simulink model "CommandePontComplet"  (R2025a)
settings: Solver=ode23t  StartTime=0.0  StopTime=5  RelTol=1e-3
libraries: spsSeriesRLCBranchLib x7, spsDiodeLib x4, spsMosfetLib x4, spsDCVoltageSourceLib x2, spsCurrentMeasurementLib x1, spsLinearTransformerLib x1, spsVoltageMeasurementLib x1, sps_lib x1
settings Model: Creator=logar  LastModifiedBy=hassan

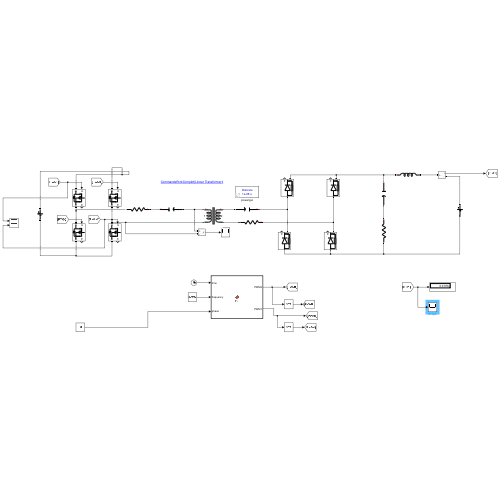
[thumbnail: Simulink's stored preview of the top-level diagram]
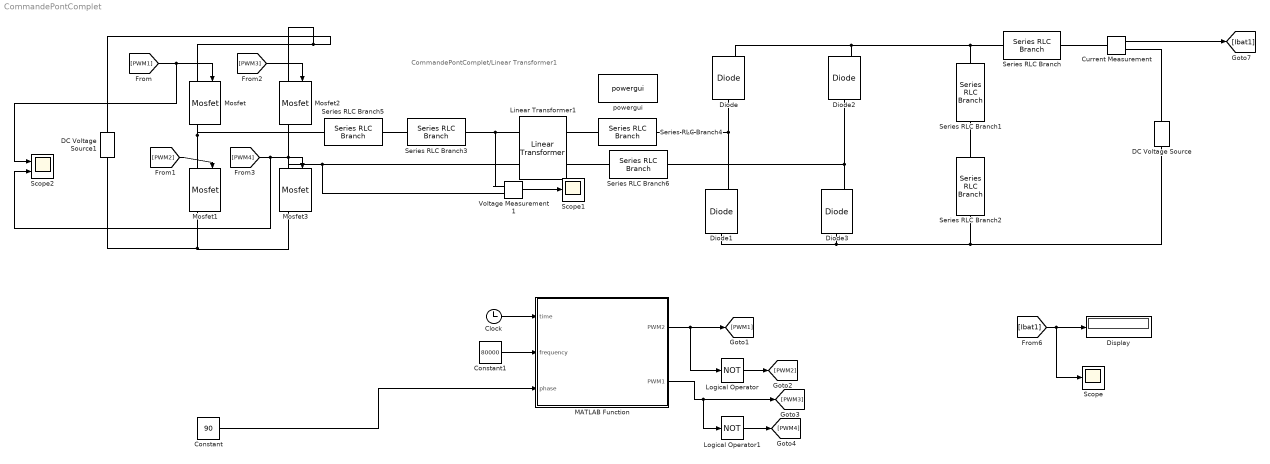
== system CommandePontComplet ==
  note: CommandePontComplet/Linear Transformer1
  Clock : Clock
  Constant : Constant  Value=90
  Constant1 : Constant  Value=80000
  Current Measurement : spsCurrentMeasurementLib/Current Measurement  PhasorSimulation=off  OutputType=Complex  PSBequivalent=0
  DC Voltage Source : spsDCVoltageSourceLib/DC Voltage Source  Amplitude=48  Measurements=None
  DC Voltage Source1 : spsDCVoltageSourceLib/DC Voltage Source  Amplitude=400  Measurements=None
  Diode{,1..3} (4 alike) : spsDiodeLib/Diode  Ron=0.001  Lon=0  Vf=0.8  IC=0  UseSnubber=0  Rs=500  Cs=250e-9  Measurements=on
  Display : Display
  Linear Transformer1 : spsLinearTransformerLib/Linear Transformer  UNITS=SI  NominalPower=[ 2000 80e3 ]  winding1=[400 4.3218e-09 0.00089501]  winding2=[70 7.938e-10 0.000338]  ThreeWindings=off  winding3=[3.15e+05 0.7938 0.084225]  RmLm=[1.0805e+06 2866.1]  Measurements=None  DataType=on
  Logical Operator : Logic  Operator=NOT  AllPortsSameDT=off  OutDataTypeStr=boolean
  Logical Operator1 : Logic  Operator=NOT  AllPortsSameDT=off  OutDataTypeStr=boolean
  MATLAB Function : MATLAB Function  TreatAsAtomicUnit=on
  Mosfet{,1..3} (4 alike) : spsMosfetLib/Mosfet  Ron=0.1  Lon=0  Rd=0.01  Vfd=0  IC=0  Rs=1e5  Cs=inf  Measurements=on
  Scope : Scope
      settings: ActiveDisplayYMinimum=-0.00099507474157943879  ActiveDisplayYMaximum=0.040324566346598756
  Scope1 : Scope
      settings: ActiveDisplayYMinimum=-402.56471596665705  ActiveDisplayYMaximum=404.97381059399561
  Scope2 : Scope  NumInputPorts=2
      settings: ActiveDisplayYMinimum=-0.025124580830577781  ActiveDisplayYMaximum=1.019798521825793  DataLoggingVariableName=ScopeData2
  Series RLC Branch : spsSeriesRLCBranchLib/Series RLC Branch  LConnTagsString=__new0  RConnTagsString=__new0  BranchType=L  Resistance=1  Inductance=40e-6  SetiL0=off  InitialCurrent=0  Capacitance=1e-6  Setx0=off  InitialVoltage=0  Measurements=None
  Series RLC Branch1 : spsSeriesRLCBranchLib/Series RLC Branch  LConnTagsString=__new0  RConnTagsString=__new0  BranchType=C  Resistance=1  Inductance=1e-3  SetiL0=off  InitialCurrent=0  Capacitance=200e-6  Setx0=off  InitialVoltage=0  Measurements=None
  Series RLC Branch2 : spsSeriesRLCBranchLib/Series RLC Branch  LConnTagsString=__new0  RConnTagsString=__new0  BranchType=R  Resistance=10e-3  Inductance=1e-3  SetiL0=off  InitialCurrent=0  Capacitance=1e-6  Setx0=off  InitialVoltage=0  Measurements=None
  Series RLC Branch3 : spsSeriesRLCBranchLib/Series RLC Branch  LConnTagsString=__new0  RConnTagsString=__new0  BranchType=C  Resistance=1  Inductance=1e-3  SetiL0=off  InitialCurrent=0  Capacitance=100e-6  Setx0=off  InitialVoltage=0  Measurements=None
  Series RLC Branch4 : spsSeriesRLCBranchLib/Series RLC Branch  LConnTagsString=__new0  RConnTagsString=__new0  BranchType=C  Resistance=1  Inductance=1e-3  SetiL0=off  InitialCurrent=0  Capacitance=47e-6  Setx0=off  InitialVoltage=0  Measurements=None
  Series RLC Branch5 : spsSeriesRLCBranchLib/Series RLC Branch  LConnTagsString=__new0  RConnTagsString=__new0  BranchType=R  Resistance=0.05  Inductance=1e-3  SetiL0=off  InitialCurrent=0  Capacitance=1e-6  Setx0=off  InitialVoltage=0  Measurements=None
  Series RLC Branch6 : spsSeriesRLCBranchLib/Series RLC Branch  LConnTagsString=__new0  RConnTagsString=__new0  BranchType=R  Resistance=50  Inductance=1e-3  SetiL0=off  InitialCurrent=0  Capacitance=1e-6  Setx0=off  InitialVoltage=0  Measurements=None
  Voltage Measurement1 : spsVoltageMeasurementLib/Voltage Measurement  PhasorSimulation=off  OutputType=Complex  PSBequivalent=0
  powergui : sps_lib/powergui  Priority=1  SimulationMode=Discrete  SampleTime=1e-8  frequency=60  Iterations=50  frequencyindice=0  Pbase=100e6  ErrMax=1e-4  UnitsV=kV  UnitsW=MW  buscounter=0  FunctionMessages=off  echomessages=off  EnableUseOfTLC=off  CurrentSourceSwitches=off  DisableSnubberDevices=off  DisableRonSwitches=off  DisableVfSwitches=off  DisplayEquations=off  AutomaticDiscreteSolvers=off  SolverType=Tustin/Backward Euler (TBE)  Interpol=off  ExternalGateDelay=off  methode=off  Ts=100  x0status=blocks  SPID=on  SwTol=0  HookPort=off  NonlinearTolerance=1e-4  nMaxIteration=100  ContinueOnMaxIteration=off  RestoreLinks=warning  ResistiveCurrentMeasurement=off  Frange=[0:2:500]  Ylog=off  Xlog=on  ShowGrid=off  save=off  variable=ZData  structure=0  ZoomFFT=off  StartTime=0.0  cycles=1  DisplayStyle=1  fundamental=60  FreqAxis=off  MaxFrequency=1000  frequencyindicesteady=1  RmsSteady=1  display=off
  wires:
  [PWM1] -> Scope2/1, Mosfet/1
  [PWM3] -> Mosfet2/1
  [PWM2] -> Mosfet1/1
  [PWM4] -> Scope2/2, Mosfet3/1
  Constant1/1 -> MATLAB Function/2(frequency)
  Clock/1 -> MATLAB Function/1(time)
  MATLAB Function/1(PWM2) -> Logical Operator/1, [PWM1]
  Logical Operator/1 -> [PWM2]
  MATLAB Function/2(PWM1) -> Logical Operator1/1, [PWM3]
  Logical Operator1/1 -> [PWM4]
  Voltage Measurement1/1 -> Scope1/1
  Current Measurement/1 -> [Ibat1]
  [Ibat1] -> Scope/1, Display/1
  Constant/1 -> MATLAB Function/3(phase)
  connections:
  Mosfet/RConn1 -- Series RLC Branch5/RConn1 -- Mosfet1/LConn1
  Mosfet2/RConn1 -- Linear Transformer1/LConn2 -- Voltage Measurement1/LConn2 -- Mosfet3/LConn1
  Mosfet2/LConn1 -- Mosfet/LConn1 -- DC Voltage Source1/RConn1
  Mosfet3/RConn1 -- DC Voltage Source1/LConn1 -- Mosfet1/RConn1
  Diode1/RConn1 -- Series RLC Branch4/LConn1 -- Diode/LConn1
  Diode3/RConn1 -- Diode2/LConn1 -- Series RLC Branch6/LConn1
  Diode2/RConn1 -- Series RLC Branch1/LConn1 -- Series RLC Branch/LConn1 -- Diode/RConn1
  Diode1/LConn1 -- DC Voltage Source/LConn1 -- Series RLC Branch2/RConn1 -- Diode3/LConn1
  Series RLC Branch/RConn1 -- Current Measurement/LConn1
  Voltage Measurement1/LConn1 -- Linear Transformer1/LConn1 -- Series RLC Branch3/RConn1
  Series RLC Branch2/LConn1 -- Series RLC Branch1/RConn1
  Series RLC Branch6/RConn1 -- Linear Transformer1/RConn2
  Series RLC Branch3/LConn1 -- Series RLC Branch5/LConn1
  Linear Transformer1/RConn1 -- Series RLC Branch4/RConn1
  DC Voltage Source/RConn1 -- Current Measurement/RConn1

== matlab function CommandePontComplet/MATLAB Function ==
  data: time input; PWM2 output; frequency input; phase input; PWM1 output
function [PWM2, PWM1] = fcn (time, frequency, phase)
Tswitching = 1/frequency;
PWM1 =0;
PWM2 =0;
y1 = mod (time, Tswitching) ;
if y1 < Tswitching/2
    PWM1 = 1;
end
t_phi = Tswitching*phase/360;
y2 = mod (time+t_phi, Tswitching) ;
if y2 < Tswitching/2
    PWM2 = 1;
end
